simulink model "ep10_25_1"  (R2018a)
settings: Solver=VariableStepAuto  StartTime=0.0  StopTime=10.0  RelTol=1e-3
settings Model: Creator=zheny  LastModifiedBy=zheny

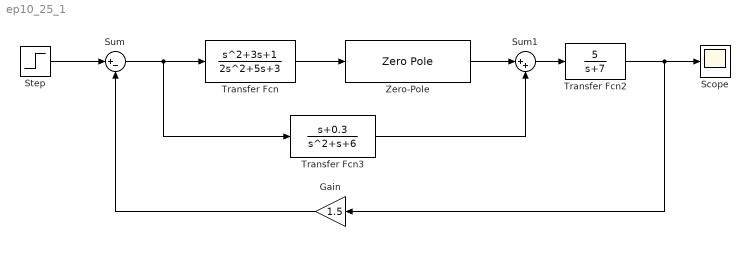
== system ep10_25_1 ==
  Gain : Gain  Gain=1.5
  Scope : Scope
  Step : Step  SampleTime=0
  Sum : Sum  Inputs=|+-
  Sum1 : Sum  Inputs=|++
  Transfer Fcn : TransferFcn  Numerator=[1 3 1]  Denominator=[2 5 3]
  Transfer Fcn2 : TransferFcn  Numerator=[5]  Denominator=[1 7]
  Transfer Fcn3 : TransferFcn  Numerator=[1 0.3]  Denominator=[1 1 6]
  Zero-Pole : ZeroPole  Zeros=-1  Poles=[-2 -10]  Gain=2
  wires:
  Step/1 -> Sum/1
  Sum/1 -> Transfer Fcn3/1, Transfer Fcn/1
  Transfer Fcn/1 -> Zero-Pole/1
  Zero-Pole/1 -> Sum1/1
  Sum1/1 -> Transfer Fcn2/1
  Transfer Fcn2/1 -> Scope/1, Gain/1
  Transfer Fcn3/1 -> Sum1/2
  Gain/1 -> Sum/2
